simulink model "task3"  (R2022b)
settings: Solver=FixedStepAuto  StartTime=0.0  StopTime=50  RelTol=1e-8
undefined symbols (not defined in the file): A, B, C, x0
settings Model: Creator=anton  LastModifiedBy=anton
settings DataIOCC: ExternalInput=data

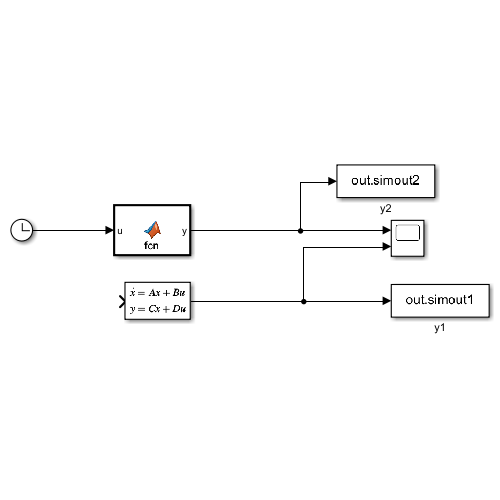
[thumbnail: Simulink's stored preview of the top-level diagram]
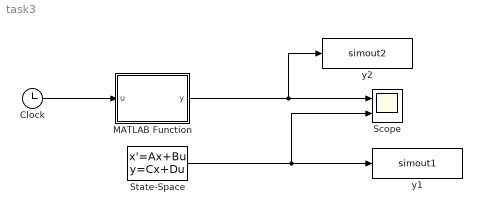
== system task3 ==
  Clock : Clock
  MATLAB Function : MATLAB Function  TreatAsAtomicUnit=on
  Scope : Scope  NumInputPorts=2
  State-Space : StateSpace  A=A  B=B  C=C  D=0  InitialCondition=x0
  y1 : ToWorkspace  VariableName=simout1  SaveFormat=Timeseries  SampleTime=-1
  y2 : ToWorkspace  VariableName=simout2  SaveFormat=Timeseries  SampleTime=-1
  wires:
  State-Space/1 -> Scope/2, y1/1
  MATLAB Function/1(y) -> y2/1, Scope/1
  Clock/1 -> MATLAB Function/1(u)

== matlab function task3/MATLAB Function ==
  data: u input; y output
function y = fcn(u)

y = cos(-2*u) + exp(6*u)*cos(5*u);
